simulink model "akh_rev_project"  (R2020b)
settings: Solver=ode45  StartTime=0.0  StopTime=10  FixedStep=Ts_Power  RelTol=1e-3  AbsTol=1e-2
InitFcn:
  | Fnom = 50;        % Hz
  | 
  | Fc = 27*Fnom;   % (Hz)
  | Ts_Power = 1/(Fc*100);
  | Ts_Control = Ts_Power*10;
values from neighbouring files (symbols this model uses):
  Ts = 1/fs    (= 1e-05)    [PE_46.m]    (also in disc_sim.m = 1; mass_spring_damper_model.m = 0.1)
undefined symbols (not defined in the file or in its folder): D1, D11, Delta, DiscIntNeverNeededParam, j, magnitude
libraries: powerlib x146, powerlib_meascontrol x90, simulink x2, re_lib x1
(part 7 of 8)

== system akh_rev_project/VSC Controller Station 1/Discrete VSC Controller /Outer Active-Reactive Power and Voltage Loop/Active_Power_Control/Int_regulator (type 1) ==
  note: Reset states when enabling
  note: Integral Regulator
      | (Type 1)
  Ord : Inport
  Meas : Inport  Port=2
  freeze : Inport  Port=3
  Enable (Reset) : EnablePort  StatesWhenEnabling=reset  PropagateVarSize=During execution
  Add : Sum
  Add1 : Sum
  Constant7 : Constant  Value=0.0
  Discrete-Time Integrator : DiscreteIntegrator  IntegratorMethod=Integration: Trapezoidal  gainval=Ki  InitialCondition=IC_i  SampleTime=Ts  LimitOutput=on  UpperSaturationLimit=max_i  LowerSaturationLimit=min_i  ICPrevOutput=DiscIntNeverNeededParam  ICPrevScaledInput=DiscIntNeverNeededParam
      settings: AttributesFormatString=Gain=%<gainval>\nMin=%<LowerSaturationLimit>\nMax=%<UpperSaturationLimit>
  Kf : Gain  Gain=Kf
      settings: AttributesFormatString=Gain=%<Gain>
  Saturation : Saturate  UpperLimit=max_out  LowerLimit=min_out
      settings: AttributesFormatString=Min=%<LowerLimit>\nMax=%<UpperLimit>
  Subtract : Sum  Inputs=+-
  Sum2 : Sum  Inputs=|+-  SaturateOnIntegerOverflow=on
  Switch : Switch  Criteria=u2 > Threshold  SaturateOnIntegerOverflow=on
  Unit Delay : UnitDelay  SampleTime=Ts_Control  HasFrameUpgradeWarning=on
      settings: AttributesFormatString=IC=%<InitialCondition>
  Out : Outport  VectorParamsAs1DForOutWhenUnconnected=off
  wires:
  Kf/1 -> Unit Delay/1
  Subtract/1 -> Switch/3
  Meas/1 -> Subtract/2
  Switch/1 -> Add/1
  Constant7/1 -> Switch/1
  freeze/1 -> Switch/2
  Discrete-Time Integrator/1 -> Add1/2
  Add1/1 -> Sum2/2, Saturation/1
  Sum2/1 -> Kf/1
  Ord/1 -> Subtract/1, Add1/1
  Add/1 -> Discrete-Time Integrator/1
  Unit Delay/1 -> Add/2
  Saturation/1 -> Sum2/1, Out/1

== system akh_rev_project/VSC Controller Station 1/Discrete VSC Controller /Outer Active-Reactive Power and Voltage Loop/Active_Power_Control/Ramping ==
  note: Output is reset to zero when the ramp is not enabled
  note: Ramping
  enable_ramp : Inport
  Pref : Inport  Port=2
  Constant12 : Constant  Value=Ramp_apc
  Logical Operator7 : Logic  Operator=NOT  AllPortsSameDT=off
  Rate Limiter with external rates & reset (discrete) IC:0 : Subsystem  mask(Rate of Change Limiter){ic=0, st=Ts_Control}
      mask prompts: ic "Initial condition (pu):"; st "Sample time (s):"
      mask help: Limit rising and falling rates of signal. When the input (R) is true the output is reset to the input (In). Rates are in p.u./s for up and -p.u./s for down.
      mask Display: disp('                Rate\n               Limiter')
  Switch : Switch  Criteria=u2 > Threshold  SaturateOnIntegerOverflow=on
  zero : Constant  Value=0.0
  Pref_ramp : Outport  VectorParamsAs1DForOutWhenUnconnected=off
  wires:
  Logical Operator7/1 -> Rate Limiter with external rates & reset (discrete) IC:0/4(R)
  Switch/1 -> Rate Limiter with external rates & reset (discrete) IC:0/1(In)
  zero/1 -> Switch/3
  Pref/1 -> Switch/1
  enable_ramp/1 -> Logical Operator7/1, Switch/2
  Constant12/1 -> Rate Limiter with external rates & reset (discrete) IC:0/3(down_rate), Rate Limiter with external rates & reset (discrete) IC:0/2(up_rate)
  Rate Limiter with external rates & reset (discrete) IC:0/1(" ") -> Pref_ramp/1

== system akh_rev_project/VSC Controller Station 1/Discrete VSC Controller /Outer Active-Reactive Power and Voltage Loop/Current_Reference_Limitation/Double click here for  info ==
  note: Power System Simulation laboratory (IREQ)
  note: Current Reference Limitation
  note: The subsystem limits the amplitude of phase current of the fundamental component to the rated current
      | of the converter.
  note: Power Control Mode
  note: DC Voltage Control Mode
  note: In power control mode, equal scaling is applied to the active and reactive power reference when a limit is imposed.
  note: In DC voltage control mode, higher priority is given to the active power when a limit is imposed.

== system akh_rev_project/VSC Controller Station 1/Discrete VSC Controller /Outer Active-Reactive Power and Voltage Loop/DC_Voltage_Control/PI_regulator (type 2) ==
  note: Regulator PI
      | (Type 2)
  Ord : Inport
  Meas : Inport  Port=2
  Add : Sum
  Add1 : Sum
  Discrete-Time Integrator : DiscreteIntegrator  IntegratorMethod=Integration: Trapezoidal  gainval=Ki  InitialCondition=i_ic  SampleTime=Ts  LimitOutput=on  UpperSaturationLimit=max_i  LowerSaturationLimit=min_i  ICPrevOutput=DiscIntNeverNeededParam  ICPrevScaledInput=DiscIntNeverNeededParam
      settings: AttributesFormatString=Gain=%<gainval>\nMin=%<LowerSaturationLimit>\nMax=%<UpperSaturationLimit>
  Kf : Gain  Gain=Kf
      settings: AttributesFormatString=Gain=%<Gain>
  Kp : Gain  Gain=Kp
      settings: AttributesFormatString=Gain=%<Gain>
  Saturation : Saturate  UpperLimit=max_out  LowerLimit=min_out
      settings: AttributesFormatString=Min=%<LowerLimit>\nMax=%<UpperLimit>
  Subtract : Sum  Inputs=+-
  Sum2 : Sum  Inputs=|+-  SaturateOnIntegerOverflow=on
  Unit Delay : UnitDelay  SampleTime=Ts_Control  HasFrameUpgradeWarning=on
      settings: AttributesFormatString=IC=%<InitialCondition>
  Out : Outport  VectorParamsAs1DForOutWhenUnconnected=off
  wires:
  Kp/1 -> Add1/1
  Sum2/1 -> Kf/1
  Subtract/1 -> Add/1, Kp/1
  Saturation/1 -> Sum2/1, Out/1
  Unit Delay/1 -> Add/2
  Add/1 -> Discrete-Time Integrator/1
  Ord/1 -> Subtract/1
  Kf/1 -> Unit Delay/1
  Add1/1 -> Saturation/1, Sum2/2
  Discrete-Time Integrator/1 -> Add1/2
  Meas/1 -> Subtract/2

== system akh_rev_project/VSC Controller Station 1/Discrete VSC Controller /Outer Active-Reactive Power and Voltage Loop/Reactive_Power_Control/AC Voltage Control Override  ==
  note: Reset states when enabling
  note: Override Regulator
  note: Active when input (In) is outside its range [min_in, max_in] otherwise the output goes back to zero
  In : Inport
  Enable (reset) : EnablePort  StatesWhenEnabling=reset  PropagateVarSize=During execution
  Add : Sum
  Constant1 : Constant  Value=max_in
  Constant2 : Constant  Value=min_in
  Constant3 : Constant  Value=Kp
  Discrete-Time Integrator1 : DiscreteIntegrator  IntegratorMethod=Integration: Trapezoidal  gainval=Ki  InitialCondition=IC_i  SampleTime=Ts  LimitOutput=on  UpperSaturationLimit=0  LowerSaturationLimit=min_out_lim  ICPrevOutput=DiscIntNeverNeededParam  ICPrevScaledInput=DiscIntNeverNeededParam
      settings: AttributesFormatString=Gain=%<gainval>\nMin=%<LowerSaturationLimit>\nMax=%<UpperSaturationLimit>
  Discrete-Time Integrator2 : DiscreteIntegrator  IntegratorMethod=Integration: Trapezoidal  gainval=Ki  InitialCondition=IC_i  SampleTime=Ts  LimitOutput=on  UpperSaturationLimit=max_out_lim  LowerSaturationLimit=0  ICPrevOutput=DiscIntNeverNeededParam  ICPrevScaledInput=DiscIntNeverNeededParam
      settings: AttributesFormatString=Gain=%<gainval>\nMin=%<LowerSaturationLimit>\nMax=%<UpperSaturationLimit>
  Product : Product  RndMeth=Zero
  Saturation : Saturate  UpperLimit=0  LowerLimit=min_out_lim
      settings: AttributesFormatString=Min=%<LowerLimit>\nMax=%<UpperLimit>
  Saturation1 : Saturate  UpperLimit=max_out_lim  LowerLimit=0
      settings: AttributesFormatString=Min=%<LowerLimit>\nMax=%<UpperLimit>
  Saturation2 : Saturate  UpperLimit=max_out_lim  LowerLimit=min_out_lim
      settings: AttributesFormatString=Min=%<LowerLimit>\nMax=%<UpperLimit>
  Subtract : Sum  Inputs=+-
  Subtract1 : Sum  Inputs=-+
  Sum2 : Sum  Inputs=+++  SaturateOnIntegerOverflow=on
  Out : Outport  VectorParamsAs1DForOutWhenUnconnected=off
  wires:
  Constant2/1 -> Subtract1/2
  Constant1/1 -> Subtract/1
  Discrete-Time Integrator2/1 -> Sum2/3  "positive"
  Discrete-Time Integrator1/1 -> Sum2/2  "negative"
  Product/1 -> Sum2/1
  Saturation1/1 -> Add/2
  Saturation/1 -> Add/1
  Add/1 -> Product/2
  Constant3/1 -> Product/1
  In/1 -> Subtract1/1, Subtract/2
  Subtract/1 -> Discrete-Time Integrator1/1, Saturation/1
  Subtract1/1 -> Saturation1/1, Discrete-Time Integrator2/1
  Sum2/1 -> Saturation2/1
  Saturation2/1 -> Out/1

== system akh_rev_project/VSC Controller Station 1/Discrete VSC Controller /Outer Active-Reactive Power and Voltage Loop/Reactive_Power_Control/Freeze_integrator ==
  note: Freeze Integrator
  note: Low AC voltage level
  U_meas : Inport
  Constant8 : Constant  Value=V_level_rpc
  Relational Operator : RelationalOperator  Operator=<=  RndMeth=Nearest
  Freeze : Outport  VectorParamsAs1DForOutWhenUnconnected=off
  wires:
  U_meas/1 -> Relational Operator/1
  Relational Operator/1 -> Freeze/1
  Constant8/1 -> Relational Operator/2

== system akh_rev_project/VSC Controller Station 1/Discrete VSC Controller /Outer Active-Reactive Power and Voltage Loop/Reactive_Power_Control/Int_regulator (type 1) ==
  note: Reset states when enabling
  note: Integral Regulator
      | (Type 1)
  Ord : Inport
  Meas : Inport  Port=2
  freeze : Inport  Port=3
  Enable (Reset) : EnablePort  StatesWhenEnabling=reset  PropagateVarSize=During execution
  Add : Sum
  Add1 : Sum
  Constant7 : Constant  Value=0.0
  Discrete-Time Integrator : DiscreteIntegrator  IntegratorMethod=Integration: Trapezoidal  gainval=Ki  InitialCondition=IC_i  SampleTime=Ts  LimitOutput=on  UpperSaturationLimit=max_i  LowerSaturationLimit=min_i  ICPrevOutput=DiscIntNeverNeededParam  ICPrevScaledInput=DiscIntNeverNeededParam
      settings: AttributesFormatString=Gain=%<gainval>\nMin=%<LowerSaturationLimit>\nMax=%<UpperSaturationLimit>
  Kf : Gain  Gain=Kf
      settings: AttributesFormatString=Gain=%<Gain>
  Saturation : Saturate  UpperLimit=max_out  LowerLimit=min_out
      settings: AttributesFormatString=Min=%<LowerLimit>\nMax=%<UpperLimit>
  Subtract : Sum  Inputs=+-
  Sum2 : Sum  Inputs=|+-  SaturateOnIntegerOverflow=on
  Switch : Switch  Criteria=u2 > Threshold  SaturateOnIntegerOverflow=on
  Unit Delay : UnitDelay  SampleTime=Ts_Control  HasFrameUpgradeWarning=on
      settings: AttributesFormatString=IC=%<InitialCondition>
  Out : Outport  VectorParamsAs1DForOutWhenUnconnected=off
  wires:
  Kf/1 -> Unit Delay/1
  Subtract/1 -> Switch/3
  Meas/1 -> Subtract/2
  Switch/1 -> Add/1
  Constant7/1 -> Switch/1
  freeze/1 -> Switch/2
  Discrete-Time Integrator/1 -> Add1/2
  Add1/1 -> Sum2/2, Saturation/1
  Sum2/1 -> Kf/1
  Ord/1 -> Subtract/1, Add1/1
  Add/1 -> Discrete-Time Integrator/1
  Unit Delay/1 -> Add/2
  Saturation/1 -> Sum2/1, Out/1

== system akh_rev_project/VSC Controller Station 2/Discrete VSC Controller /Clark Transformations/CLARK  with Rotating reference/CLARK ==
  note: CLARK transformation
  abc : Inport
  Enable (held) : EnablePort  PropagateVarSize=During execution
  abc to Alpha-Beta-Zero : powerlib_meascontrol/Transformations/abc to Alpha-Beta-Zero
  AB0 : Outport  VectorParamsAs1DForOutWhenUnconnected=off
  wires:
  abc to Alpha-Beta-Zero/1 -> AB0/1
  abc/1 -> abc to Alpha-Beta-Zero/1

== system akh_rev_project/VSC Controller Station 2/Discrete VSC Controller /Clark Transformations/CLARK  with Rotating reference/CLARK_lag ==
  note: CLARK transformation - YD1
  abc : Inport
  Enable : EnablePort  PropagateVarSize=During execution
  Fcn1 : Fcn  Expr=(-u[1] - u[3] + 2*u[2] )/3
  Fcn2 : Fcn  Expr=(u[1]-u[3])/sqrt(3)
  Fcn3 : Fcn  Expr=0
  Mux : Mux  Inputs=3
  AB0 : Outport  VectorParamsAs1DForOutWhenUnconnected=off
  wires:
  Fcn2/1 -> Mux/1
  abc/1 -> Fcn1/1, Fcn3/1, Fcn2/1
  Fcn1/1 -> Mux/2
  Fcn3/1 -> Mux/3
  Mux/1 -> AB0/1

== system akh_rev_project/VSC Controller Station 2/Discrete VSC Controller /Clark Transformations/CLARK  with Rotating reference/CLARK_lead ==
  note: CLARK transformation - YD11
  abc : Inport
  Enable : EnablePort  PropagateVarSize=During execution
  Fcn1 : Fcn  Expr=(u[1] + u[2] - 2*u[3] )/3
  Fcn2 : Fcn  Expr=(u[1]-u[2])/sqrt(3)
  Fcn3 : Fcn  Expr=0
  Mux : Mux  Inputs=3
  AB0 : Outport  VectorParamsAs1DForOutWhenUnconnected=off
  wires:
  Mux/1 -> AB0/1
  Fcn3/1 -> Mux/3
  Fcn1/1 -> Mux/2
  abc/1 -> Fcn2/1, Fcn3/1, Fcn1/1
  Fcn2/1 -> Mux/1

== system akh_rev_project/VSC Controller Station 2/Discrete VSC Controller /Clark Transformations/CLARK  with Rotating reference1/CLARK ==
  note: CLARK transformation
  abc : Inport
  Enable (held) : EnablePort  PropagateVarSize=During execution
  abc to Alpha-Beta-Zero : powerlib_meascontrol/Transformations/abc to Alpha-Beta-Zero
  AB0 : Outport  VectorParamsAs1DForOutWhenUnconnected=off
  wires:
  abc to Alpha-Beta-Zero/1 -> AB0/1
  abc/1 -> abc to Alpha-Beta-Zero/1

== system akh_rev_project/VSC Controller Station 2/Discrete VSC Controller /Clark Transformations/CLARK  with Rotating reference1/CLARK_lag ==
  note: CLARK transformation - YD1
  abc : Inport
  Enable : EnablePort  PropagateVarSize=During execution
  Fcn1 : Fcn  Expr=(-u[1] - u[3] + 2*u[2] )/3
  Fcn2 : Fcn  Expr=(u[1]-u[3])/sqrt(3)
  Fcn3 : Fcn  Expr=0
  Mux : Mux  Inputs=3
  AB0 : Outport  VectorParamsAs1DForOutWhenUnconnected=off
  wires:
  Fcn2/1 -> Mux/1
  abc/1 -> Fcn1/1, Fcn3/1, Fcn2/1
  Fcn1/1 -> Mux/2
  Fcn3/1 -> Mux/3
  Mux/1 -> AB0/1

== system akh_rev_project/VSC Controller Station 2/Discrete VSC Controller /Clark Transformations/CLARK  with Rotating reference1/CLARK_lead ==
  note: CLARK transformation - YD11
  abc : Inport
  Enable : EnablePort  PropagateVarSize=During execution
  Fcn1 : Fcn  Expr=(u[1] + u[2] - 2*u[3] )/3
  Fcn2 : Fcn  Expr=(u[1]-u[2])/sqrt(3)
  Fcn3 : Fcn  Expr=0
  Mux : Mux  Inputs=3
  AB0 : Outport  VectorParamsAs1DForOutWhenUnconnected=off
  wires:
  Mux/1 -> AB0/1
  Fcn3/1 -> Mux/3
  Fcn1/1 -> Mux/2
  abc/1 -> Fcn2/1, Fcn3/1, Fcn1/1
  Fcn2/1 -> Mux/1

== system akh_rev_project/VSC Controller Station 2/Discrete VSC Controller /DC Voltage Balance Control/Regulator/PI_regulator (type 2) ==
  note: Regulator PI
      | (Type 2)
  Ord : Inport
  Meas : Inport  Port=2
  Add : Sum
  Add1 : Sum
  Discrete-Time Integrator : DiscreteIntegrator  IntegratorMethod=Integration: Trapezoidal  gainval=Ki  InitialCondition=i_ic  SampleTime=Ts  LimitOutput=on  UpperSaturationLimit=max_i  LowerSaturationLimit=min_i  ICPrevOutput=DiscIntNeverNeededParam  ICPrevScaledInput=DiscIntNeverNeededParam
      settings: AttributesFormatString=Gain=%<gainval>\nMin=%<LowerSaturationLimit>\nMax=%<UpperSaturationLimit>
  Kf : Gain  Gain=Kf
      settings: AttributesFormatString=Gain=%<Gain>
  Kp : Gain  Gain=Kp
      settings: AttributesFormatString=Gain=%<Gain>
  Saturation : Saturate  UpperLimit=max_out  LowerLimit=min_out
      settings: AttributesFormatString=Min=%<LowerLimit>\nMax=%<UpperLimit>
  Subtract : Sum  Inputs=+-
  Sum2 : Sum  Inputs=|+-  SaturateOnIntegerOverflow=on
  Unit Delay : UnitDelay  SampleTime=Ts_Control  HasFrameUpgradeWarning=on
      settings: AttributesFormatString=IC=%<InitialCondition>
  Out : Outport  VectorParamsAs1DForOutWhenUnconnected=off
  wires:
  Kp/1 -> Add1/1
  Sum2/1 -> Kf/1
  Subtract/1 -> Add/1, Kp/1
  Saturation/1 -> Sum2/1, Out/1
  Unit Delay/1 -> Add/2
  Add/1 -> Discrete-Time Integrator/1
  Ord/1 -> Subtract/1
  Kf/1 -> Unit Delay/1
  Add1/1 -> Saturation/1, Sum2/2
  Discrete-Time Integrator/1 -> Add1/2
  Meas/1 -> Subtract/2

== system akh_rev_project/VSC Controller Station 2/Discrete VSC Controller /Inner Current Loop/AC_Current_Control/PI_regulator 1 ==
  note: Regulator PI
      | (Type 2)
  Ord : Inport
  Meas : Inport  Port=2
  Add : Sum
  Add1 : Sum
  Discrete-Time Integrator : DiscreteIntegrator  IntegratorMethod=Integration: Trapezoidal  gainval=Ki  InitialCondition=i_ic  SampleTime=Ts  LimitOutput=on  UpperSaturationLimit=max_i  LowerSaturationLimit=min_i  ICPrevOutput=DiscIntNeverNeededParam  ICPrevScaledInput=DiscIntNeverNeededParam
      settings: AttributesFormatString=Gain=%<gainval>\nMin=%<LowerSaturationLimit>\nMax=%<UpperSaturationLimit>
  Kf : Gain  Gain=Kf
      settings: AttributesFormatString=Gain=%<Gain>
  Kp : Gain  Gain=Kp
      settings: AttributesFormatString=Gain=%<Gain>
  Saturation : Saturate  UpperLimit=max_out  LowerLimit=min_out
      settings: AttributesFormatString=Min=%<LowerLimit>\nMax=%<UpperLimit>
  Subtract : Sum  Inputs=+-
  Sum2 : Sum  Inputs=|+-  SaturateOnIntegerOverflow=on
  Unit Delay : UnitDelay  SampleTime=Ts_Control  HasFrameUpgradeWarning=on
      settings: AttributesFormatString=IC=%<InitialCondition>
  Out : Outport  VectorParamsAs1DForOutWhenUnconnected=off
  wires:
  Kp/1 -> Add1/1
  Sum2/1 -> Kf/1
  Subtract/1 -> Add/1, Kp/1
  Saturation/1 -> Sum2/1, Out/1
  Unit Delay/1 -> Add/2
  Add/1 -> Discrete-Time Integrator/1
  Ord/1 -> Subtract/1
  Kf/1 -> Unit Delay/1
  Add1/1 -> Saturation/1, Sum2/2
  Discrete-Time Integrator/1 -> Add1/2
  Meas/1 -> Subtract/2

== system akh_rev_project/VSC Controller Station 2/Discrete VSC Controller /Inner Current Loop/AC_Current_Control/PI_regulator 2 ==
  note: Regulator PI
      | (Type 2)
  Ord : Inport
  Meas : Inport  Port=2
  Add : Sum
  Add1 : Sum
  Discrete-Time Integrator : DiscreteIntegrator  IntegratorMethod=Integration: Trapezoidal  gainval=Ki  InitialCondition=i_ic  SampleTime=Ts  LimitOutput=on  UpperSaturationLimit=max_i  LowerSaturationLimit=min_i  ICPrevOutput=DiscIntNeverNeededParam  ICPrevScaledInput=DiscIntNeverNeededParam
      settings: AttributesFormatString=Gain=%<gainval>\nMin=%<LowerSaturationLimit>\nMax=%<UpperSaturationLimit>
  Kf : Gain  Gain=Kf
      settings: AttributesFormatString=Gain=%<Gain>
  Kp : Gain  Gain=Kp
      settings: AttributesFormatString=Gain=%<Gain>
  Saturation : Saturate  UpperLimit=max_out  LowerLimit=min_out
      settings: AttributesFormatString=Min=%<LowerLimit>\nMax=%<UpperLimit>
  Subtract : Sum  Inputs=+-
  Sum2 : Sum  Inputs=|+-  SaturateOnIntegerOverflow=on
  Unit Delay : UnitDelay  SampleTime=Ts_Control  HasFrameUpgradeWarning=on
      settings: AttributesFormatString=IC=%<InitialCondition>
  Out : Outport  VectorParamsAs1DForOutWhenUnconnected=off
  wires:
  Kp/1 -> Add1/1
  Sum2/1 -> Kf/1
  Subtract/1 -> Add/1, Kp/1
  Saturation/1 -> Sum2/1, Out/1
  Unit Delay/1 -> Add/2
  Add/1 -> Discrete-Time Integrator/1
  Ord/1 -> Subtract/1
  Kf/1 -> Unit Delay/1
  Add1/1 -> Saturation/1, Sum2/2
  Discrete-Time Integrator/1 -> Add1/2
  Meas/1 -> Subtract/2

== system akh_rev_project/VSC Controller Station 2/Discrete VSC Controller /Outer Active-Reactive Power and Voltage Loop/Active_Power_Control/DC Voltage Control Override ==
  note: Reset states when enabling
  note: Override Regulator
  note: Active when input (In) is outside its range [min_in, max_in] otherwise the output goes back to zero
  In : Inport
  Enable (reset) : EnablePort  StatesWhenEnabling=reset  PropagateVarSize=During execution
  Add : Sum
  Constant1 : Constant  Value=max_in
  Constant2 : Constant  Value=min_in
  Constant3 : Constant  Value=Kp
  Discrete-Time Integrator1 : DiscreteIntegrator  IntegratorMethod=Integration: Trapezoidal  gainval=Ki  InitialCondition=IC_i  SampleTime=Ts  LimitOutput=on  UpperSaturationLimit=0  LowerSaturationLimit=min_out_lim  ICPrevOutput=DiscIntNeverNeededParam  ICPrevScaledInput=DiscIntNeverNeededParam
      settings: AttributesFormatString=Gain=%<gainval>\nMin=%<LowerSaturationLimit>\nMax=%<UpperSaturationLimit>
  Discrete-Time Integrator2 : DiscreteIntegrator  IntegratorMethod=Integration: Trapezoidal  gainval=Ki  InitialCondition=IC_i  SampleTime=Ts  LimitOutput=on  UpperSaturationLimit=max_out_lim  LowerSaturationLimit=0  ICPrevOutput=DiscIntNeverNeededParam  ICPrevScaledInput=DiscIntNeverNeededParam
      settings: AttributesFormatString=Gain=%<gainval>\nMin=%<LowerSaturationLimit>\nMax=%<UpperSaturationLimit>
  Product : Product  RndMeth=Zero
  Saturation : Saturate  UpperLimit=0  LowerLimit=min_out_lim
      settings: AttributesFormatString=Min=%<LowerLimit>\nMax=%<UpperLimit>
  Saturation1 : Saturate  UpperLimit=max_out_lim  LowerLimit=0
      settings: AttributesFormatString=Min=%<LowerLimit>\nMax=%<UpperLimit>
  Saturation2 : Saturate  UpperLimit=max_out_lim  LowerLimit=min_out_lim
      settings: AttributesFormatString=Min=%<LowerLimit>\nMax=%<UpperLimit>
  Subtract : Sum  Inputs=+-
  Subtract1 : Sum  Inputs=-+
  Sum2 : Sum  Inputs=+++  SaturateOnIntegerOverflow=on
  Out : Outport  VectorParamsAs1DForOutWhenUnconnected=off
  wires:
  Constant2/1 -> Subtract1/2
  Constant1/1 -> Subtract/1
  Discrete-Time Integrator2/1 -> Sum2/3  "positive"
  Discrete-Time Integrator1/1 -> Sum2/2  "negative"
  Product/1 -> Sum2/1
  Saturation1/1 -> Add/2
  Saturation/1 -> Add/1
  Add/1 -> Product/2
  Constant3/1 -> Product/1
  In/1 -> Subtract1/1, Subtract/2
  Subtract/1 -> Discrete-Time Integrator1/1, Saturation/1
  Subtract1/1 -> Saturation1/1, Discrete-Time Integrator2/1
  Sum2/1 -> Saturation2/1
  Saturation2/1 -> Out/1

== system akh_rev_project/VSC Controller Station 2/Discrete VSC Controller /Outer Active-Reactive Power and Voltage Loop/Active_Power_Control/Freeze_integrator ==
  note: Low AC voltage level
  note: Freeze Integrator
  U_meas : Inport
  Constant8 : Constant  Value=V_level_apc
  Relational Operator : RelationalOperator  Operator=<=  RndMeth=Nearest
  Freeze : Outport  VectorParamsAs1DForOutWhenUnconnected=off
  wires:
  Constant8/1 -> Relational Operator/2
  Relational Operator/1 -> Freeze/1
  U_meas/1 -> Relational Operator/1

== system akh_rev_project/VSC Controller Station 2/Discrete VSC Controller /Outer Active-Reactive Power and Voltage Loop/Active_Power_Control/Int_regulator (type 1) ==
  note: Reset states when enabling
  note: Integral Regulator
      | (Type 1)
  Ord : Inport
  Meas : Inport  Port=2
  freeze : Inport  Port=3
  Enable (Reset) : EnablePort  StatesWhenEnabling=reset  PropagateVarSize=During execution
  Add : Sum
  Add1 : Sum
  Constant7 : Constant  Value=0.0
  Discrete-Time Integrator : DiscreteIntegrator  IntegratorMethod=Integration: Trapezoidal  gainval=Ki  InitialCondition=IC_i  SampleTime=Ts  LimitOutput=on  UpperSaturationLimit=max_i  LowerSaturationLimit=min_i  ICPrevOutput=DiscIntNeverNeededParam  ICPrevScaledInput=DiscIntNeverNeededParam
      settings: AttributesFormatString=Gain=%<gainval>\nMin=%<LowerSaturationLimit>\nMax=%<UpperSaturationLimit>
  Kf : Gain  Gain=Kf
      settings: AttributesFormatString=Gain=%<Gain>
  Saturation : Saturate  UpperLimit=max_out  LowerLimit=min_out
      settings: AttributesFormatString=Min=%<LowerLimit>\nMax=%<UpperLimit>
  Subtract : Sum  Inputs=+-
  Sum2 : Sum  Inputs=|+-  SaturateOnIntegerOverflow=on
  Switch : Switch  Criteria=u2 > Threshold  SaturateOnIntegerOverflow=on
  Unit Delay : UnitDelay  SampleTime=Ts_Control  HasFrameUpgradeWarning=on
      settings: AttributesFormatString=IC=%<InitialCondition>
  Out : Outport  VectorParamsAs1DForOutWhenUnconnected=off
  wires:
  Kf/1 -> Unit Delay/1
  Subtract/1 -> Switch/3
  Meas/1 -> Subtract/2
  Switch/1 -> Add/1
  Constant7/1 -> Switch/1
  freeze/1 -> Switch/2
  Discrete-Time Integrator/1 -> Add1/2
  Add1/1 -> Sum2/2, Saturation/1
  Sum2/1 -> Kf/1
  Ord/1 -> Subtract/1, Add1/1
  Add/1 -> Discrete-Time Integrator/1
  Unit Delay/1 -> Add/2
  Saturation/1 -> Sum2/1, Out/1

== system akh_rev_project/VSC Controller Station 2/Discrete VSC Controller /Outer Active-Reactive Power and Voltage Loop/Active_Power_Control/Ramping ==
  note: Output is reset to zero when the ramp is not enabled
  note: Ramping
  enable_ramp : Inport
  Pref : Inport  Port=2
  Constant12 : Constant  Value=Ramp_apc
  Logical Operator7 : Logic  Operator=NOT  AllPortsSameDT=off
  Rate Limiter with external rates & reset (discrete) IC:0 : Subsystem  mask(Rate of Change Limiter){ic=0, st=Ts_Control}
      mask prompts: ic "Initial condition (pu):"; st "Sample time (s):"
      mask help: Limit rising and falling rates of signal. When the input (R) is true the output is reset to the input (In). Rates are in p.u./s for up and -p.u./s for down.
      mask Display: disp('                Rate\n               Limiter')
  Switch : Switch  Criteria=u2 > Threshold  SaturateOnIntegerOverflow=on
  zero : Constant  Value=0.0
  Pref_ramp : Outport  VectorParamsAs1DForOutWhenUnconnected=off
  wires:
  Logical Operator7/1 -> Rate Limiter with external rates & reset (discrete) IC:0/4(R)
  Switch/1 -> Rate Limiter with external rates & reset (discrete) IC:0/1(In)
  zero/1 -> Switch/3
  Pref/1 -> Switch/1
  enable_ramp/1 -> Logical Operator7/1, Switch/2
  Constant12/1 -> Rate Limiter with external rates & reset (discrete) IC:0/3(down_rate), Rate Limiter with external rates & reset (discrete) IC:0/2(up_rate)
  Rate Limiter with external rates & reset (discrete) IC:0/1(" ") -> Pref_ramp/1

== system akh_rev_project/VSC Controller Station 2/Discrete VSC Controller /Outer Active-Reactive Power and Voltage Loop/Current_Reference_Limitation/Double click here for  info ==
  note: Power System Simulation laboratory (IREQ)
  note: Current Reference Limitation
  note: The subsystem limits the amplitude of phase current of the fundamental component to the rated current
      | of the converter.
  note: Power Control Mode
  note: DC Voltage Control Mode
  note: In power control mode, equal scaling is applied to the active and reactive power reference when a limit is imposed.
  note: In DC voltage control mode, higher priority is given to the active power when a limit is imposed.

== system akh_rev_project/VSC Controller Station 2/Discrete VSC Controller /Outer Active-Reactive Power and Voltage Loop/DC_Voltage_Control/PI_regulator (type 2) ==
  note: Regulator PI
      | (Type 2)
  Ord : Inport
  Meas : Inport  Port=2
  Add : Sum
  Add1 : Sum
  Discrete-Time Integrator : DiscreteIntegrator  IntegratorMethod=Integration: Trapezoidal  gainval=Ki  InitialCondition=i_ic  SampleTime=Ts  LimitOutput=on  UpperSaturationLimit=max_i  LowerSaturationLimit=min_i  ICPrevOutput=DiscIntNeverNeededParam  ICPrevScaledInput=DiscIntNeverNeededParam
      settings: AttributesFormatString=Gain=%<gainval>\nMin=%<LowerSaturationLimit>\nMax=%<UpperSaturationLimit>
  Kf : Gain  Gain=Kf
      settings: AttributesFormatString=Gain=%<Gain>
  Kp : Gain  Gain=Kp
      settings: AttributesFormatString=Gain=%<Gain>
  Saturation : Saturate  UpperLimit=max_out  LowerLimit=min_out
      settings: AttributesFormatString=Min=%<LowerLimit>\nMax=%<UpperLimit>
  Subtract : Sum  Inputs=+-
  Sum2 : Sum  Inputs=|+-  SaturateOnIntegerOverflow=on
  Unit Delay : UnitDelay  SampleTime=Ts_Control  HasFrameUpgradeWarning=on
      settings: AttributesFormatString=IC=%<InitialCondition>
  Out : Outport  VectorParamsAs1DForOutWhenUnconnected=off
  wires:
  Kp/1 -> Add1/1
  Sum2/1 -> Kf/1
  Subtract/1 -> Add/1, Kp/1
  Saturation/1 -> Sum2/1, Out/1
  Unit Delay/1 -> Add/2
  Add/1 -> Discrete-Time Integrator/1
  Ord/1 -> Subtract/1
  Kf/1 -> Unit Delay/1
  Add1/1 -> Saturation/1, Sum2/2
  Discrete-Time Integrator/1 -> Add1/2
  Meas/1 -> Subtract/2

== system akh_rev_project/VSC Controller Station 2/Discrete VSC Controller /Outer Active-Reactive Power and Voltage Loop/Reactive_Power_Control/AC Voltage Control Override  ==
  note: Reset states when enabling
  note: Override Regulator
  note: Active when input (In) is outside its range [min_in, max_in] otherwise the output goes back to zero
  In : Inport
  Enable (reset) : EnablePort  StatesWhenEnabling=reset  PropagateVarSize=During execution
  Add : Sum
  Constant1 : Constant  Value=max_in
  Constant2 : Constant  Value=min_in
  Constant3 : Constant  Value=Kp
  Discrete-Time Integrator1 : DiscreteIntegrator  IntegratorMethod=Integration: Trapezoidal  gainval=Ki  InitialCondition=IC_i  SampleTime=Ts  LimitOutput=on  UpperSaturationLimit=0  LowerSaturationLimit=min_out_lim  ICPrevOutput=DiscIntNeverNeededParam  ICPrevScaledInput=DiscIntNeverNeededParam
      settings: AttributesFormatString=Gain=%<gainval>\nMin=%<LowerSaturationLimit>\nMax=%<UpperSaturationLimit>
  Discrete-Time Integrator2 : DiscreteIntegrator  IntegratorMethod=Integration: Trapezoidal  gainval=Ki  InitialCondition=IC_i  SampleTime=Ts  LimitOutput=on  UpperSaturationLimit=max_out_lim  LowerSaturationLimit=0  ICPrevOutput=DiscIntNeverNeededParam  ICPrevScaledInput=DiscIntNeverNeededParam
      settings: AttributesFormatString=Gain=%<gainval>\nMin=%<LowerSaturationLimit>\nMax=%<UpperSaturationLimit>
  Product : Product  RndMeth=Zero
  Saturation : Saturate  UpperLimit=0  LowerLimit=min_out_lim
      settings: AttributesFormatString=Min=%<LowerLimit>\nMax=%<UpperLimit>
  Saturation1 : Saturate  UpperLimit=max_out_lim  LowerLimit=0
      settings: AttributesFormatString=Min=%<LowerLimit>\nMax=%<UpperLimit>
  Saturation2 : Saturate  UpperLimit=max_out_lim  LowerLimit=min_out_lim
      settings: AttributesFormatString=Min=%<LowerLimit>\nMax=%<UpperLimit>
  Subtract : Sum  Inputs=+-
  Subtract1 : Sum  Inputs=-+
  Sum2 : Sum  Inputs=+++  SaturateOnIntegerOverflow=on
  Out : Outport  VectorParamsAs1DForOutWhenUnconnected=off
  wires:
  Constant2/1 -> Subtract1/2
  Constant1/1 -> Subtract/1
  Discrete-Time Integrator2/1 -> Sum2/3  "positive"
  Discrete-Time Integrator1/1 -> Sum2/2  "negative"
  Product/1 -> Sum2/1
  Saturation1/1 -> Add/2
  Saturation/1 -> Add/1
  Add/1 -> Product/2
  Constant3/1 -> Product/1
  In/1 -> Subtract1/1, Subtract/2
  Subtract/1 -> Discrete-Time Integrator1/1, Saturation/1
  Subtract1/1 -> Saturation1/1, Discrete-Time Integrator2/1
  Sum2/1 -> Saturation2/1
  Saturation2/1 -> Out/1

== system akh_rev_project/VSC Controller Station 2/Discrete VSC Controller /Outer Active-Reactive Power and Voltage Loop/Reactive_Power_Control/Freeze_integrator ==
  note: Freeze Integrator
  note: Low AC voltage level
  U_meas : Inport
  Constant8 : Constant  Value=V_level_rpc
  Relational Operator : RelationalOperator  Operator=<=  RndMeth=Nearest
  Freeze : Outport  VectorParamsAs1DForOutWhenUnconnected=off
  wires:
  U_meas/1 -> Relational Operator/1
  Relational Operator/1 -> Freeze/1
  Constant8/1 -> Relational Operator/2

== system akh_rev_project/VSC Controller Station 2/Discrete VSC Controller /Outer Active-Reactive Power and Voltage Loop/Reactive_Power_Control/Int_regulator (type 1) ==
  note: Reset states when enabling
  note: Integral Regulator
      | (Type 1)
  Ord : Inport
  Meas : Inport  Port=2
  freeze : Inport  Port=3
  Enable (Reset) : EnablePort  StatesWhenEnabling=reset  PropagateVarSize=During execution
  Add : Sum
  Add1 : Sum
  Constant7 : Constant  Value=0.0
  Discrete-Time Integrator : DiscreteIntegrator  IntegratorMethod=Integration: Trapezoidal  gainval=Ki  InitialCondition=IC_i  SampleTime=Ts  LimitOutput=on  UpperSaturationLimit=max_i  LowerSaturationLimit=min_i  ICPrevOutput=DiscIntNeverNeededParam  ICPrevScaledInput=DiscIntNeverNeededParam
      settings: AttributesFormatString=Gain=%<gainval>\nMin=%<LowerSaturationLimit>\nMax=%<UpperSaturationLimit>
  Kf : Gain  Gain=Kf
      settings: AttributesFormatString=Gain=%<Gain>
  Saturation : Saturate  UpperLimit=max_out  LowerLimit=min_out
      settings: AttributesFormatString=Min=%<LowerLimit>\nMax=%<UpperLimit>
  Subtract : Sum  Inputs=+-
  Sum2 : Sum  Inputs=|+-  SaturateOnIntegerOverflow=on
  Switch : Switch  Criteria=u2 > Threshold  SaturateOnIntegerOverflow=on
  Unit Delay : UnitDelay  SampleTime=Ts_Control  HasFrameUpgradeWarning=on
      settings: AttributesFormatString=IC=%<InitialCondition>
  Out : Outport  VectorParamsAs1DForOutWhenUnconnected=off
  wires:
  Kf/1 -> Unit Delay/1
  Subtract/1 -> Switch/3
  Meas/1 -> Subtract/2
  Switch/1 -> Add/1
  Constant7/1 -> Switch/1
  freeze/1 -> Switch/2
  Discrete-Time Integrator/1 -> Add1/2
  Add1/1 -> Sum2/2, Saturation/1
  Sum2/1 -> Kf/1
  Ord/1 -> Subtract/1, Add1/1
  Add/1 -> Discrete-Time Integrator/1
  Unit Delay/1 -> Add/2
  Saturation/1 -> Sum2/1, Out/1

== system akh_rev_project/AC System 1/Plant 2 MVA/Plant & Motor Protection/AC Current Protection/Current Measurement/magnitude ==
  In1 : Inport
  Complex to Real-Imag : ComplexToRealImag
  Fourier1 : Subsystem  mask(Fourier analyser){f1=Freq, n=0}
      mask prompts: f1 "Fundamental frequency f1 (Hz):"; n "Harmonic n (0=DC; 1=fundamental; 2=2nd harm;  ...) :"
      mask help: The Fourier block performs a Fourier analysis of the input signal over a running window of one cycle of the fundamental frequency. First and second outputs return respectively the magnitude and phase (degrees) of the harmonic component specified.
      mask init:
      | k=2-(n==0);
      mask Help: helpview(psbhelp)
  Fourier2 : Subsystem  mask(Fourier analyser){f1=Freq, n=0}
      mask prompts: f1 "Fundamental frequency f1 (Hz):"; n "Harmonic n (0=DC; 1=fundamental; 2=2nd harm;  ...) :"
      mask help: The Fourier block performs a Fourier analysis of the input signal over a running window of one cycle of the fundamental frequency. First and second outputs return respectively the magnitude and phase (degrees) of the harmonic component specified.
      mask init:
      | k=2-(n==0);
      mask Help: helpview(psbhelp)
  Math Function : Math  Operator=hypot  SignedPower=on  SaturateOnIntegerOverflow=on
  Terminator : Terminator
  Terminator1 : Terminator
  Out1 : Outport  VectorParamsAs1DForOutWhenUnconnected=off
  wires:
  In1/1 -> Complex to Real-Imag/1
  Math Function/1 -> Out1/1
  Fourier2/1(magnitude) -> Math Function/2
  Fourier1/1(magnitude) -> Math Function/1
  Fourier2/2(angle) -> Terminator1/1
  Fourier1/2(angle) -> Terminator/1
  Complex to Real-Imag/2 -> Fourier2/1(signal)
  Complex to Real-Imag/1 -> Fourier1/1(signal)

== system akh_rev_project/AC System 1/Plant 2 MVA/Plant & Motor Protection/AC Current Protection/Current Measurement/magnitude1 ==
  In1 : Inport
  Complex to Real-Imag : ComplexToRealImag
  Fourier1 : Subsystem  mask(Fourier analyser){f1=Freq, n=0}
      mask prompts: f1 "Fundamental frequency f1 (Hz):"; n "Harmonic n (0=DC; 1=fundamental; 2=2nd harm;  ...) :"
      mask help: The Fourier block performs a Fourier analysis of the input signal over a running window of one cycle of the fundamental frequency. First and second outputs return respectively the magnitude and phase (degrees) of the harmonic component specified.
      mask init:
      | k=2-(n==0);
      mask Help: helpview(psbhelp)
  Fourier2 : Subsystem  mask(Fourier analyser){f1=Freq, n=0}
      mask prompts: f1 "Fundamental frequency f1 (Hz):"; n "Harmonic n (0=DC; 1=fundamental; 2=2nd harm;  ...) :"
      mask help: The Fourier block performs a Fourier analysis of the input signal over a running window of one cycle of the fundamental frequency. First and second outputs return respectively the magnitude and phase (degrees) of the harmonic component specified.
      mask init:
      | k=2-(n==0);
      mask Help: helpview(psbhelp)
  Math Function : Math  Operator=hypot  SignedPower=on  SaturateOnIntegerOverflow=on
  Terminator : Terminator
  Terminator1 : Terminator
  Out1 : Outport  VectorParamsAs1DForOutWhenUnconnected=off
  wires:
  Complex to Real-Imag/1 -> Fourier1/1(signal)
  Complex to Real-Imag/2 -> Fourier2/1(signal)
  Fourier1/2(angle) -> Terminator/1
  Fourier2/2(angle) -> Terminator1/1
  Fourier1/1(magnitude) -> Math Function/1
  Fourier2/1(magnitude) -> Math Function/2
  Math Function/1 -> Out1/1
  In1/1 -> Complex to Real-Imag/1

== system akh_rev_project/AC System 1/Plant 2 MVA/Plant & Motor Protection/AC Voltage Protection/Voltage Measurement/magnitude ==
  In1 : Inport
  Complex to Real-Imag : ComplexToRealImag
  Fourier1 : Subsystem  mask(Fourier analyser){f1=Freq, n=0}
      mask prompts: f1 "Fundamental frequency f1 (Hz):"; n "Harmonic n (0=DC; 1=fundamental; 2=2nd harm;  ...) :"
      mask help: The Fourier block performs a Fourier analysis of the input signal over a running window of one cycle of the fundamental frequency. First and second outputs return respectively the magnitude and phase (degrees) of the harmonic component specified.
      mask init:
      | k=2-(n==0);
      mask Help: helpview(psbhelp)
  Fourier2 : Subsystem  mask(Fourier analyser){f1=Freq, n=0}
      mask prompts: f1 "Fundamental frequency f1 (Hz):"; n "Harmonic n (0=DC; 1=fundamental; 2=2nd harm;  ...) :"
      mask help: The Fourier block performs a Fourier analysis of the input signal over a running window of one cycle of the fundamental frequency. First and second outputs return respectively the magnitude and phase (degrees) of the harmonic component specified.
      mask init:
      | k=2-(n==0);
      mask Help: helpview(psbhelp)
  Math Function : Math  Operator=hypot  SignedPower=on  SaturateOnIntegerOverflow=on
  Terminator : Terminator
  Terminator1 : Terminator
  Out1 : Outport  VectorParamsAs1DForOutWhenUnconnected=off
  wires:
  In1/1 -> Complex to Real-Imag/1
  Math Function/1 -> Out1/1
  Fourier2/1(magnitude) -> Math Function/2
  Fourier1/1(magnitude) -> Math Function/1
  Fourier2/2(angle) -> Terminator1/1
  Fourier1/2(angle) -> Terminator/1
  Complex to Real-Imag/2 -> Fourier2/1(signal)
  Complex to Real-Imag/1 -> Fourier1/1(signal)

== system akh_rev_project/AC System 1/Plant 2 MVA/Plant & Motor Protection/AC Voltage Protection/Voltage Measurement/magnitude1 ==
  In1 : Inport
  Complex to Real-Imag : ComplexToRealImag
  Fourier1 : Subsystem  mask(Fourier analyser){f1=Freq, n=0}
      mask prompts: f1 "Fundamental frequency f1 (Hz):"; n "Harmonic n (0=DC; 1=fundamental; 2=2nd harm;  ...) :"
      mask help: The Fourier block performs a Fourier analysis of the input signal over a running window of one cycle of the fundamental frequency. First and second outputs return respectively the magnitude and phase (degrees) of the harmonic component specified.
      mask init:
      | k=2-(n==0);
      mask Help: helpview(psbhelp)
  Fourier2 : Subsystem  mask(Fourier analyser){f1=Freq, n=0}
      mask prompts: f1 "Fundamental frequency f1 (Hz):"; n "Harmonic n (0=DC; 1=fundamental; 2=2nd harm;  ...) :"
      mask help: The Fourier block performs a Fourier analysis of the input signal over a running window of one cycle of the fundamental frequency. First and second outputs return respectively the magnitude and phase (degrees) of the harmonic component specified.
      mask init:
      | k=2-(n==0);
      mask Help: helpview(psbhelp)
  Math Function : Math  Operator=hypot  SignedPower=on  SaturateOnIntegerOverflow=on
  Terminator : Terminator
  Terminator1 : Terminator
  Out1 : Outport  VectorParamsAs1DForOutWhenUnconnected=off
  wires:
  Complex to Real-Imag/1 -> Fourier1/1(signal)
  Complex to Real-Imag/2 -> Fourier2/1(signal)
  Fourier1/2(angle) -> Terminator/1
  Fourier2/2(angle) -> Terminator1/1
  Fourier1/1(magnitude) -> Math Function/1
  Fourier2/1(magnitude) -> Math Function/2
  Math Function/1 -> Out1/1
  In1/1 -> Complex to Real-Imag/1

== system akh_rev_project/AC System 1/Plant 2 MVA/Plant & Motor Protection/AC Voltage Protection/Voltage Measurement/magnitude2 ==
  In1 : Inport
  Complex to Real-Imag : ComplexToRealImag
  Fourier1 : Subsystem  mask(Fourier analyser){f1=Freq, n=0}
      mask prompts: f1 "Fundamental frequency f1 (Hz):"; n "Harmonic n (0=DC; 1=fundamental; 2=2nd harm;  ...) :"
      mask help: The Fourier block performs a Fourier analysis of the input signal over a running window of one cycle of the fundamental frequency. First and second outputs return respectively the magnitude and phase (degrees) of the harmonic component specified.
      mask init:
      | k=2-(n==0);
      mask Help: helpview(psbhelp)
  Fourier2 : Subsystem  mask(Fourier analyser){f1=Freq, n=0}
      mask prompts: f1 "Fundamental frequency f1 (Hz):"; n "Harmonic n (0=DC; 1=fundamental; 2=2nd harm;  ...) :"
      mask help: The Fourier block performs a Fourier analysis of the input signal over a running window of one cycle of the fundamental frequency. First and second outputs return respectively the magnitude and phase (degrees) of the harmonic component specified.
      mask init:
      | k=2-(n==0);
      mask Help: helpview(psbhelp)
  Math Function : Math  Operator=hypot  SignedPower=on  SaturateOnIntegerOverflow=on
  Terminator : Terminator
  Terminator1 : Terminator
  Out1 : Outport  VectorParamsAs1DForOutWhenUnconnected=off
  wires:
  In1/1 -> Complex to Real-Imag/1
  Math Function/1 -> Out1/1
  Fourier2/1(magnitude) -> Math Function/2
  Fourier1/1(magnitude) -> Math Function/1
  Fourier2/2(angle) -> Terminator1/1
  Fourier1/2(angle) -> Terminator/1
  Complex to Real-Imag/2 -> Fourier2/1(signal)
  Complex to Real-Imag/1 -> Fourier1/1(signal)

== system akh_rev_project/AC System 1/Wind Turbine Protection/Protection System/AC Current Protection/Current Measurement/magnitude ==
  In1 : Inport
  Complex to Real-Imag : ComplexToRealImag
  Fourier1 : Subsystem  mask(Fourier analyser){f1=Freq, n=0}
      mask prompts: f1 "Fundamental frequency f1 (Hz):"; n "Harmonic n (0=DC; 1=fundamental; 2=2nd harm;  ...) :"
      mask help: The Fourier block performs a Fourier analysis of the input signal over a running window of one cycle of the fundamental frequency. First and second outputs return respectively the magnitude and phase (degrees) of the harmonic component specified.
      mask init:
      | k=2-(n==0);
      mask Help: helpview(psbhelp)
  Fourier2 : Subsystem  mask(Fourier analyser){f1=Freq, n=0}
      mask prompts: f1 "Fundamental frequency f1 (Hz):"; n "Harmonic n (0=DC; 1=fundamental; 2=2nd harm;  ...) :"
      mask help: The Fourier block performs a Fourier analysis of the input signal over a running window of one cycle of the fundamental frequency. First and second outputs return respectively the magnitude and phase (degrees) of the harmonic component specified.
      mask init:
      | k=2-(n==0);
      mask Help: helpview(psbhelp)
  Math Function : Math  Operator=hypot  SignedPower=on  SaturateOnIntegerOverflow=on
  Terminator : Terminator
  Terminator1 : Terminator
  Out1 : Outport  VectorParamsAs1DForOutWhenUnconnected=off
  wires:
  Complex to Real-Imag/1 -> Fourier1/1(signal)
  Complex to Real-Imag/2 -> Fourier2/1(signal)
  Fourier1/2(angle) -> Terminator/1
  Fourier2/2(angle) -> Terminator1/1
  Fourier1/1(magnitude) -> Math Function/1
  Fourier2/1(magnitude) -> Math Function/2
  Math Function/1 -> Out1/1
  In1/1 -> Complex to Real-Imag/1

== system akh_rev_project/AC System 1/Wind Turbine Protection/Protection System/AC Current Protection/Current Measurement/magnitude1 ==
  In1 : Inport
  Complex to Real-Imag : ComplexToRealImag
  Fourier1 : Subsystem  mask(Fourier analyser){f1=Freq, n=0}
      mask prompts: f1 "Fundamental frequency f1 (Hz):"; n "Harmonic n (0=DC; 1=fundamental; 2=2nd harm;  ...) :"
      mask help: The Fourier block performs a Fourier analysis of the input signal over a running window of one cycle of the fundamental frequency. First and second outputs return respectively the magnitude and phase (degrees) of the harmonic component specified.
      mask init:
      | k=2-(n==0);
      mask Help: helpview(psbhelp)
  Fourier2 : Subsystem  mask(Fourier analyser){f1=Freq, n=0}
      mask prompts: f1 "Fundamental frequency f1 (Hz):"; n "Harmonic n (0=DC; 1=fundamental; 2=2nd harm;  ...) :"
      mask help: The Fourier block performs a Fourier analysis of the input signal over a running window of one cycle of the fundamental frequency. First and second outputs return respectively the magnitude and phase (degrees) of the harmonic component specified.
      mask init:
      | k=2-(n==0);
      mask Help: helpview(psbhelp)
  Math Function : Math  Operator=hypot  SignedPower=on  SaturateOnIntegerOverflow=on
  Terminator : Terminator
  Terminator1 : Terminator
  Out1 : Outport  VectorParamsAs1DForOutWhenUnconnected=off
  wires:
  In1/1 -> Complex to Real-Imag/1
  Math Function/1 -> Out1/1
  Fourier2/1(magnitude) -> Math Function/2
  Fourier1/1(magnitude) -> Math Function/1
  Fourier2/2(angle) -> Terminator1/1
  Fourier1/2(angle) -> Terminator/1
  Complex to Real-Imag/2 -> Fourier2/1(signal)
  Complex to Real-Imag/1 -> Fourier1/1(signal)

== system akh_rev_project/AC System 1/Wind Turbine Protection/Protection System/AC Voltage Protection/Voltage Measurement/magnitude ==
  In1 : Inport
  Complex to Real-Imag : ComplexToRealImag
  Fourier1 : Subsystem  mask(Fourier analyser){f1=Freq, n=0}
      mask prompts: f1 "Fundamental frequency f1 (Hz):"; n "Harmonic n (0=DC; 1=fundamental; 2=2nd harm;  ...) :"
      mask help: The Fourier block performs a Fourier analysis of the input signal over a running window of one cycle of the fundamental frequency. First and second outputs return respectively the magnitude and phase (degrees) of the harmonic component specified.
      mask init:
      | k=2-(n==0);
      mask Help: helpview(psbhelp)
  Fourier2 : Subsystem  mask(Fourier analyser){f1=Freq, n=0}
      mask prompts: f1 "Fundamental frequency f1 (Hz):"; n "Harmonic n (0=DC; 1=fundamental; 2=2nd harm;  ...) :"
      mask help: The Fourier block performs a Fourier analysis of the input signal over a running window of one cycle of the fundamental frequency. First and second outputs return respectively the magnitude and phase (degrees) of the harmonic component specified.
      mask init:
      | k=2-(n==0);
      mask Help: helpview(psbhelp)
  Math Function : Math  Operator=hypot  SignedPower=on  SaturateOnIntegerOverflow=on
  Terminator : Terminator
  Terminator1 : Terminator
  Out1 : Outport  VectorParamsAs1DForOutWhenUnconnected=off
  wires:
  Complex to Real-Imag/1 -> Fourier1/1(signal)
  Complex to Real-Imag/2 -> Fourier2/1(signal)
  Fourier1/2(angle) -> Terminator/1
  Fourier2/2(angle) -> Terminator1/1
  Fourier1/1(magnitude) -> Math Function/1
  Fourier2/1(magnitude) -> Math Function/2
  Math Function/1 -> Out1/1
  In1/1 -> Complex to Real-Imag/1

== system akh_rev_project/AC System 1/Wind Turbine Protection/Protection System/AC Voltage Protection/Voltage Measurement/magnitude1 ==
  In1 : Inport
  Complex to Real-Imag : ComplexToRealImag
  Fourier1 : Subsystem  mask(Fourier analyser){f1=Freq, n=0}
      mask prompts: f1 "Fundamental frequency f1 (Hz):"; n "Harmonic n (0=DC; 1=fundamental; 2=2nd harm;  ...) :"
      mask help: The Fourier block performs a Fourier analysis of the input signal over a running window of one cycle of the fundamental frequency. First and second outputs return respectively the magnitude and phase (degrees) of the harmonic component specified.
      mask init:
      | k=2-(n==0);
      mask Help: helpview(psbhelp)
  Fourier2 : Subsystem  mask(Fourier analyser){f1=Freq, n=0}
      mask prompts: f1 "Fundamental frequency f1 (Hz):"; n "Harmonic n (0=DC; 1=fundamental; 2=2nd harm;  ...) :"
      mask help: The Fourier block performs a Fourier analysis of the input signal over a running window of one cycle of the fundamental frequency. First and second outputs return respectively the magnitude and phase (degrees) of the harmonic component specified.
      mask init:
      | k=2-(n==0);
      mask Help: helpview(psbhelp)
  Math Function : Math  Operator=hypot  SignedPower=on  SaturateOnIntegerOverflow=on
  Terminator : Terminator
  Terminator1 : Terminator
  Out1 : Outport  VectorParamsAs1DForOutWhenUnconnected=off
  wires:
  In1/1 -> Complex to Real-Imag/1
  Math Function/1 -> Out1/1
  Fourier2/1(magnitude) -> Math Function/2
  Fourier1/1(magnitude) -> Math Function/1
  Fourier2/2(angle) -> Terminator1/1
  Fourier1/2(angle) -> Terminator/1
  Complex to Real-Imag/2 -> Fourier2/1(signal)
  Complex to Real-Imag/1 -> Fourier1/1(signal)

== system akh_rev_project/AC System 1/Wind Turbine Protection/Protection System/AC Voltage Protection/Voltage Measurement/magnitude2 ==
  In1 : Inport
  Complex to Real-Imag : ComplexToRealImag
  Fourier1 : Subsystem  mask(Fourier analyser){f1=Freq, n=0}
      mask prompts: f1 "Fundamental frequency f1 (Hz):"; n "Harmonic n (0=DC; 1=fundamental; 2=2nd harm;  ...) :"
      mask help: The Fourier block performs a Fourier analysis of the input signal over a running window of one cycle of the fundamental frequency. First and second outputs return respectively the magnitude and phase (degrees) of the harmonic component specified.
      mask init:
      | k=2-(n==0);
      mask Help: helpview(psbhelp)
  Fourier2 : Subsystem  mask(Fourier analyser){f1=Freq, n=0}
      mask prompts: f1 "Fundamental frequency f1 (Hz):"; n "Harmonic n (0=DC; 1=fundamental; 2=2nd harm;  ...) :"
      mask help: The Fourier block performs a Fourier analysis of the input signal over a running window of one cycle of the fundamental frequency. First and second outputs return respectively the magnitude and phase (degrees) of the harmonic component specified.
      mask init:
      | k=2-(n==0);
      mask Help: helpview(psbhelp)
  Math Function : Math  Operator=hypot  SignedPower=on  SaturateOnIntegerOverflow=on
  Terminator : Terminator
  Terminator1 : Terminator
  Out1 : Outport  VectorParamsAs1DForOutWhenUnconnected=off
  wires:
  Complex to Real-Imag/1 -> Fourier1/1(signal)
  Complex to Real-Imag/2 -> Fourier2/1(signal)
  Fourier1/2(angle) -> Terminator/1
  Fourier2/2(angle) -> Terminator1/1
  Fourier1/1(magnitude) -> Math Function/1
  Fourier2/1(magnitude) -> Math Function/2
  Math Function/1 -> Out1/1
  In1/1 -> Complex to Real-Imag/1
